simulink model "Compass_Servo_Model"  (Simulink 7.1)
settings: Solver=ode45  StartTime=0.0  StopTime=10.0  RelTol=1e-3
undefined symbols (not defined in the file or in its folder): schedule
libraries: truetime x4, simulink x1
settings Model: Creator=jporter  LastModifiedBy=jporter

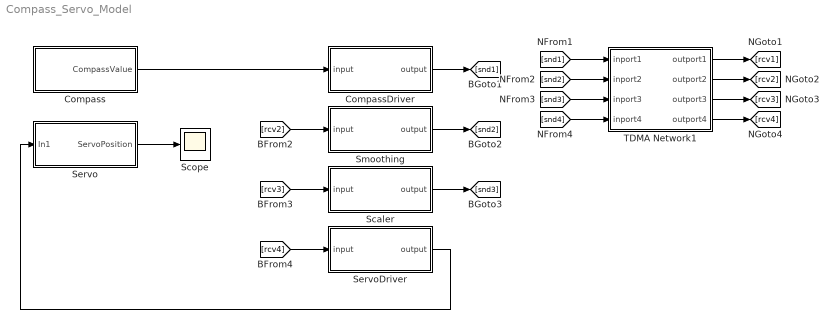
== system Compass_Servo_Model ==
  Compass : Subsystem
  CompassDriver : Subsystem
  Scaler : Subsystem
  Scope : Scope
      settings: YMin=30  YMax=180
  Servo : Subsystem
  ServoDriver : Subsystem
  Smoothing : Subsystem
  TDMA Network1 : Subsystem
  wires:
  Servo/1(ServoPosition) -> Scope/1
  TDMA Network1/1(outport1) -> [rcv1]
  [snd1] -> TDMA Network1/1(inport1)
  TDMA Network1/2(outport2) -> [rcv2]
  [snd2] -> TDMA Network1/2(inport2)
  TDMA Network1/3(outport3) -> [rcv3]
  [snd3] -> TDMA Network1/3(inport3)
  TDMA Network1/4(outport4) -> [rcv4]
  [snd4] -> TDMA Network1/4(inport4)
  CompassDriver/1(output) -> [snd1]
  [rcv2] -> Smoothing/1(input)
  Smoothing/1(output) -> [snd2]
  [rcv3] -> Scaler/1(input)
  Scaler/1(output) -> [snd3]
  [rcv4] -> ServoDriver/1(input)
  Compass/1(CompassValue) -> CompassDriver/1(input)
  ServoDriver/1(output) -> Servo/1(In1)

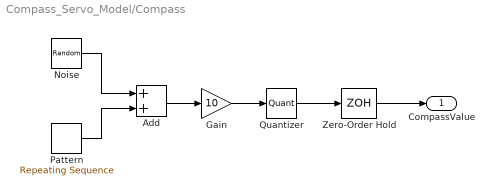
== system Compass_Servo_Model/Compass ==
  Add : Sum  OutDataType=sfix(16)  OutScaling=2^-10
  Gain : Gain  Gain=10  ParameterDataType=sfix(16)  ParameterScaling=2^0  OutDataType=sfix(16)  OutScaling=2^0
  Noise : RandomNumber  SampleTime=0
  Pattern : simulink/Sources/Repeating Sequence  SystemSampleTime=-1  rep_seq_t=[0 10]  rep_seq_y=[0 360]
  Quantizer : Quantizer  QuantizationInterval=1
  Zero-Order Hold : ZeroOrderHold  SampleTime=1/8
  CompassValue : Outport  OutDataType=sfix(16)  OutScaling=2^0
  wires:
  Noise/1 -> Add/1
  Pattern/1 -> Add/2
  Zero-Order Hold/1 -> CompassValue/1
  Add/1 -> Gain/1
  Gain/1 -> Quantizer/1
  Quantizer/1 -> Zero-Order Hold/1

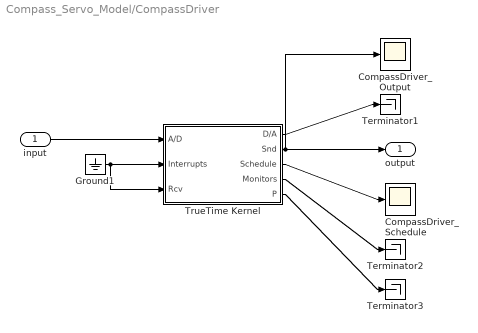
== system Compass_Servo_Model/CompassDriver ==
  input : Inport
  CompassDriver_Output : Scope
      settings: DataFormat=Array
  CompassDriver_Schedule : Scope
      settings: DataFormat=Array
  Ground1 : Ground
  Terminator1 : Terminator
  Terminator2 : Terminator
  Terminator3 : Terminator
  TrueTime Kernel : Subsystem  mask{sfun=Generic_Init, args=schedule, clockdrift=0, clockoffset=0}
      mask prompts: sfun "Name of init function (MEX or MATLAB)"; args "Init function argument"; clockdrift "Clock drift"; clockoffset "Clock offset"
  output : Outport
  wires:
  input/1 -> TrueTime Kernel/1(A/D)
  Ground1/1 -> TrueTime Kernel/3(Rcv), TrueTime Kernel/2(Interrupts)
  TrueTime Kernel/2(Snd) -> output/1, CompassDriver_Output/1
  TrueTime Kernel/1(D/A) -> Terminator1/1
  TrueTime Kernel/3(Schedule) -> CompassDriver_Schedule/1
  TrueTime Kernel/4(Monitors) -> Terminator2/1
  TrueTime Kernel/5(P) -> Terminator3/1

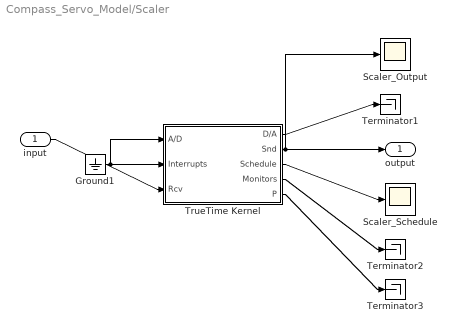
== system Compass_Servo_Model/Scaler ==
  input : Inport
  Ground1 : Ground
  Scaler_Output : Scope
      settings: DataFormat=Array
  Scaler_Schedule : Scope
      settings: DataFormat=Array
  Terminator1 : Terminator
  Terminator2 : Terminator
  Terminator3 : Terminator
  TrueTime Kernel : Subsystem  mask{sfun=Generic_Init, args=schedule, clockdrift=0, clockoffset=0}
      mask prompts: sfun "Name of init function (MEX or MATLAB)"; args "Init function argument"; clockdrift "Clock drift"; clockoffset "Clock offset"
  output : Outport
  wires:
  input/1 -> TrueTime Kernel/3(Rcv)
  Ground1/1 -> TrueTime Kernel/1(A/D), TrueTime Kernel/2(Interrupts)
  TrueTime Kernel/2(Snd) -> output/1, Scaler_Output/1
  TrueTime Kernel/1(D/A) -> Terminator1/1
  TrueTime Kernel/3(Schedule) -> Scaler_Schedule/1
  TrueTime Kernel/4(Monitors) -> Terminator2/1
  TrueTime Kernel/5(P) -> Terminator3/1

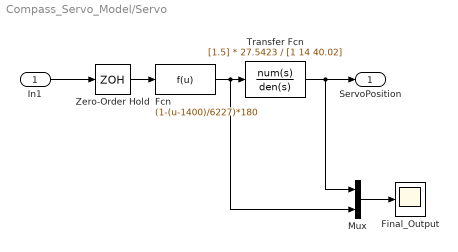
== system Compass_Servo_Model/Servo ==
  In1 : Inport  OutDataType=sfix(16)  OutScaling=2^0
  Fcn : Fcn  Expr=(1-(u-1400)/6227)*180  SampleTime=1/8
  Final_Output : Scope
      settings: YMin=20  YMax=180  SaveName=ScopeData6
  Mux : Mux  Inputs=2
  Transfer Fcn : TransferFcn  Numerator=[1.5] * 27.5423  Denominator=[1 14 40.02]
  Zero-Order Hold : ZeroOrderHold  SampleTime=1/8
  ServoPosition : Outport  OutDataType=sfix(16)  OutScaling=2^0
  wires:
  Transfer Fcn/1 -> ServoPosition/1, Mux/1
  In1/1 -> Zero-Order Hold/1
  Fcn/1 -> Mux/2, Transfer Fcn/1
  Zero-Order Hold/1 -> Fcn/1
  Mux/1 -> Final_Output/1

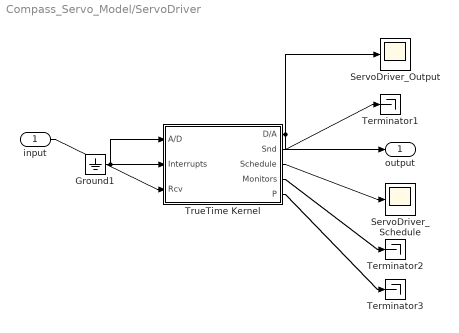
== system Compass_Servo_Model/ServoDriver ==
  input : Inport
  Ground1 : Ground
  ServoDriver_Output : Scope
      settings: DataFormat=Array
  ServoDriver_Schedule : Scope
      settings: DataFormat=Array
  Terminator1 : Terminator
  Terminator2 : Terminator
  Terminator3 : Terminator
  TrueTime Kernel : Subsystem  mask{sfun=Generic_Init, args=schedule, clockdrift=0, clockoffset=0}
      mask prompts: sfun "Name of init function (MEX or MATLAB)"; args "Init function argument"; clockdrift "Clock drift"; clockoffset "Clock offset"
  output : Outport
  wires:
  input/1 -> TrueTime Kernel/3(Rcv)
  Ground1/1 -> TrueTime Kernel/1(A/D), TrueTime Kernel/2(Interrupts)
  TrueTime Kernel/1(D/A) -> output/1, ServoDriver_Output/1
  TrueTime Kernel/2(Snd) -> Terminator1/1
  TrueTime Kernel/3(Schedule) -> ServoDriver_Schedule/1
  TrueTime Kernel/4(Monitors) -> Terminator2/1
  TrueTime Kernel/5(P) -> Terminator3/1

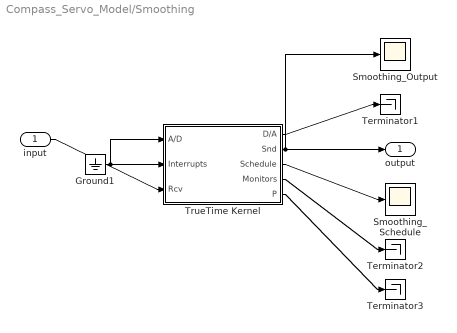
== system Compass_Servo_Model/Smoothing ==
  input : Inport
  Ground1 : Ground
  Smoothing_Output : Scope
      settings: DataFormat=Array
  Smoothing_Schedule : Scope
      settings: DataFormat=Array
  Terminator1 : Terminator
  Terminator2 : Terminator
  Terminator3 : Terminator
  TrueTime Kernel : Subsystem  mask{sfun=Generic_Init, args=schedule, clockdrift=0, clockoffset=0}
      mask prompts: sfun "Name of init function (MEX or MATLAB)"; args "Init function argument"; clockdrift "Clock drift"; clockoffset "Clock offset"
  output : Outport
  wires:
  input/1 -> TrueTime Kernel/3(Rcv)
  Ground1/1 -> TrueTime Kernel/1(A/D), TrueTime Kernel/2(Interrupts)
  TrueTime Kernel/2(Snd) -> output/1, Smoothing_Output/1
  TrueTime Kernel/1(D/A) -> Terminator1/1
  TrueTime Kernel/3(Schedule) -> Smoothing_Schedule/1
  TrueTime Kernel/4(Monitors) -> Terminator2/1
  TrueTime Kernel/5(P) -> Terminator3/1

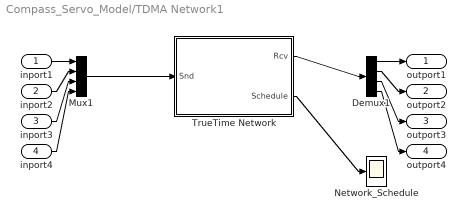
== system Compass_Servo_Model/TDMA Network1 ==
  inport1 : Inport
  inport2 : Inport  Port=2
  inport3 : Inport  Port=3
  inport4 : Inport  Port=4
  Demux1 : Demux
  Mux1 : Mux
  Network_Schedule : Scope
      settings: DataFormat=Array
  TrueTime Network : Subsystem  mask{nwtype=TDMA, nwnbr=1, nnodes=4, rate=10000000, minsize=512, lossprob=0, bandwidths=[0.5 0.5], slotsize=512, schedule=[1 2 3 4], memsize=80000, buftype=Common Buffer, overflow=Retransmit}
      mask prompts: nwtype "Network type"; nwnbr "Network number"; nnodes "Number of nodes"; rate "Data rate (bits/s)"; minsize "Minimum frame size (bits)"; lossprob "Loss probability (0-1)"; bandwidths "Bandwidth allocations"; slotsize "Slotsize (bits)"; schedule "Cyclic schedule"; memsize "Total switch memory (bits)"; buftype "Switch buffer type"; overflow "Switch overflow behavior"
      mask StyleString: popup(CSMA/CD (Ethernet)|CSMA/AMP (CAN)|Round Robin|FDMA|TDMA|Switched Ethernet),edit,edit,edit,edit,edit,edit,edit,edit,edit,popup(Common buffer|Symmetric output buffers),popup(Retransmit|Drop)
  outport1 : Outport
  outport2 : Outport  Port=2
  outport3 : Outport  Port=3
  outport4 : Outport  Port=4
  wires:
  Mux1/1 -> TrueTime Network/1(Snd)
  TrueTime Network/1(Rcv) -> Demux1/1
  TrueTime Network/2(Schedule) -> Network_Schedule/1
  Demux1/1 -> outport1/1
  inport1/1 -> Mux1/1
  Demux1/2 -> outport2/1
  inport2/1 -> Mux1/2
  Demux1/3 -> outport3/1
  inport3/1 -> Mux1/3
  Demux1/4 -> outport4/1
  inport4/1 -> Mux1/4

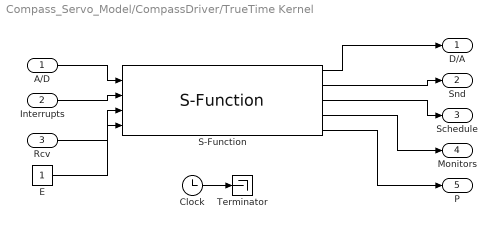
== system Compass_Servo_Model/CompassDriver/TrueTime Kernel ==
  A/D : Inport
  Interrupts : Inport  Port=2
  Rcv : Inport  Port=3
  Clock : Clock
      settings: Decimation=10
  E : Constant
  S-Function : truetime/TrueTime Kernel/S-Function
  Terminator : Terminator
  D/A : Outport
  Snd : Outport  Port=2
  Schedule : Outport  Port=3
  Monitors : Outport  Port=4
  P : Outport  Port=5
  wires:
  S-Function/5 -> P/1
  E/1 -> S-Function/4
  A/D/1 -> S-Function/1
  S-Function/2 -> Snd/1
  S-Function/1 -> D/A/1
  S-Function/3 -> Schedule/1
  S-Function/4 -> Monitors/1
  Interrupts/1 -> S-Function/2
  Rcv/1 -> S-Function/3
  Clock/1 -> Terminator/1

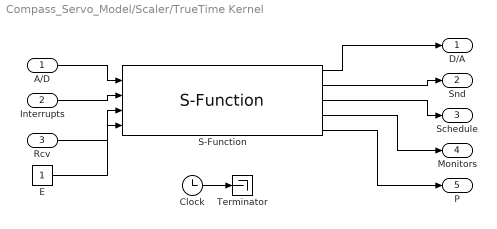
== system Compass_Servo_Model/Scaler/TrueTime Kernel ==
  A/D : Inport
  Interrupts : Inport  Port=2
  Rcv : Inport  Port=3
  Clock : Clock
      settings: Decimation=10
  E : Constant
  S-Function : truetime/TrueTime Kernel/S-Function
  Terminator : Terminator
  D/A : Outport
  Snd : Outport  Port=2
  Schedule : Outport  Port=3
  Monitors : Outport  Port=4
  P : Outport  Port=5
  wires:
  S-Function/5 -> P/1
  E/1 -> S-Function/4
  A/D/1 -> S-Function/1
  S-Function/2 -> Snd/1
  S-Function/1 -> D/A/1
  S-Function/3 -> Schedule/1
  S-Function/4 -> Monitors/1
  Interrupts/1 -> S-Function/2
  Rcv/1 -> S-Function/3
  Clock/1 -> Terminator/1

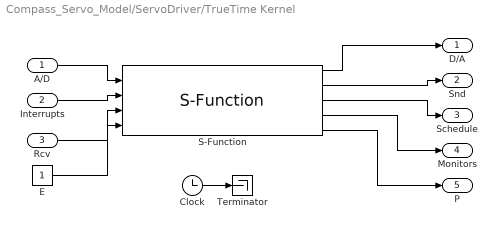
== system Compass_Servo_Model/ServoDriver/TrueTime Kernel ==
  A/D : Inport
  Interrupts : Inport  Port=2
  Rcv : Inport  Port=3
  Clock : Clock
      settings: Decimation=10
  E : Constant
  S-Function : truetime/TrueTime Kernel/S-Function
  Terminator : Terminator
  D/A : Outport
  Snd : Outport  Port=2
  Schedule : Outport  Port=3
  Monitors : Outport  Port=4
  P : Outport  Port=5
  wires:
  S-Function/5 -> P/1
  E/1 -> S-Function/4
  A/D/1 -> S-Function/1
  S-Function/2 -> Snd/1
  S-Function/1 -> D/A/1
  S-Function/3 -> Schedule/1
  S-Function/4 -> Monitors/1
  Interrupts/1 -> S-Function/2
  Rcv/1 -> S-Function/3
  Clock/1 -> Terminator/1

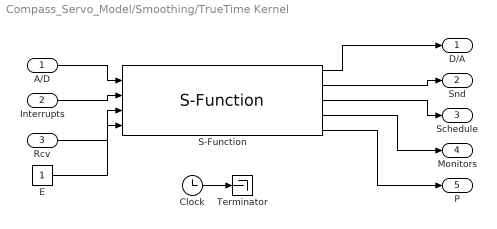
== system Compass_Servo_Model/Smoothing/TrueTime Kernel ==
  A/D : Inport
  Interrupts : Inport  Port=2
  Rcv : Inport  Port=3
  Clock : Clock
      settings: Decimation=10
  E : Constant
  S-Function : truetime/TrueTime Kernel/S-Function
  Terminator : Terminator
  D/A : Outport
  Snd : Outport  Port=2
  Schedule : Outport  Port=3
  Monitors : Outport  Port=4
  P : Outport  Port=5
  wires:
  S-Function/5 -> P/1
  E/1 -> S-Function/4
  A/D/1 -> S-Function/1
  S-Function/2 -> Snd/1
  S-Function/1 -> D/A/1
  S-Function/3 -> Schedule/1
  S-Function/4 -> Monitors/1
  Interrupts/1 -> S-Function/2
  Rcv/1 -> S-Function/3
  Clock/1 -> Terminator/1

== system Compass_Servo_Model/TDMA Network1/TrueTime Network ==
  Snd : Inport
  ttnetwork : S-Function  FunctionName=ttnetwork  Parameters=nwtype,nwnbr,nnodes,rate,minsize,lossprob,bandwidths,slotsize,schedule,memsize,buftype,overflow  EnableBusSupport=off
  Rcv : Outport
  Schedule : Outport  Port=2
  wires:
  ttnetwork/2 -> Schedule/1
  ttnetwork/1 -> Rcv/1
  Snd/1 -> ttnetwork/1
